simulink model "transmitFullSim2019a"  (R2019a)
settings: Solver=VariableStepAuto  StartTime=0.0  StopTime=0.25  RelTol=1e-3
values from neighbouring files (symbols this model uses):
  Cappr = 5.0616e-11    [transmitData.m]
  Ipr = 2.5055e-7    (= 2.5055e-07)    [transmitData.m]
  Nbps = 4    [transmitData.m]
  Rpr = 45e-3    (= 0.045)    [transmitData.m]
  Ts = 1e-8    (= 1e-08)    [transmitData.m]
libraries: rfports1 x2, commdigbbndam3 x2, commrfcorlib x1, commchan3 x1, commrandsrc3 x1, rftxlines1 x1, commsink2 x1, commutil2 x1, commrflib2 x1
settings Model: Creator=PABLO  LastModifiedBy=marekkulawik

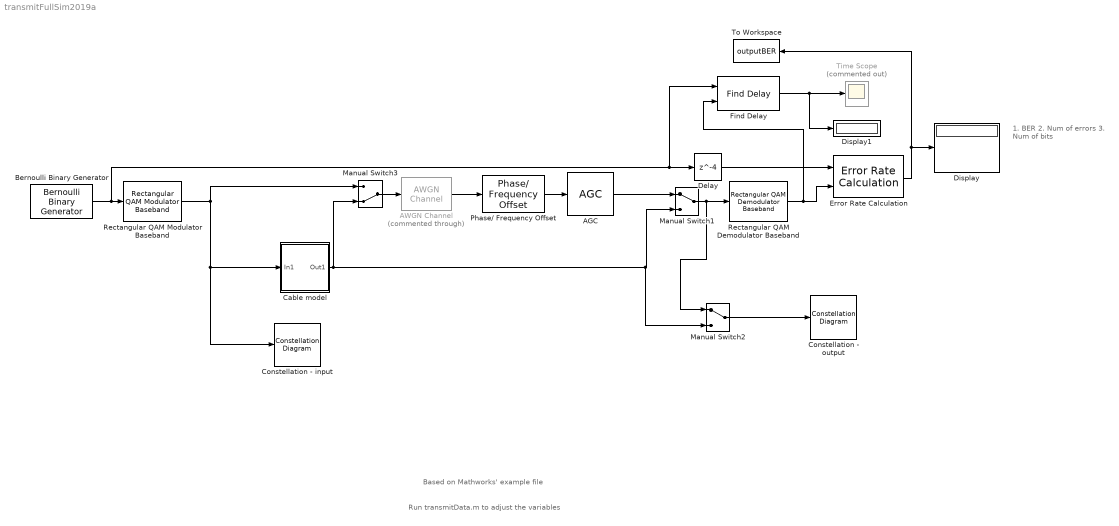
== system transmitFullSim2019a ==
  note: 1. BER
      | 2. Num of errors
      | 3. Num of bits
  note: Run transmitData.m to adjust the variables
  note: Based on Mathworks' example file
  AGC : commrfcorlib/AGC  LegacyMode=off  DetectorMethod=Rectifier  LoopMethod=Linear  UpdatePeriod=100  StepSize=0.1  AdaptationStepSize=0.001  DesiredOutputPower=1  AveragingLength=100  MaximumGain=30  MaxPowerGain=60  GainOutputPort=off  InputPowerOutputPort=off  SimulateUsing=Interpreted execution
      settings: SourceProductName=Communications Toolbox
  AWGN Channel : commchan3/AWGN Channel  Commented=through  InputProcessing=Columns as channels (frame based)  seed=54321  noiseMode="Signal to noise ratio  (SNR)"  EbNodB=EbN0  EsNodB=40  SNRdB=SNR  bitsPerSym=Nbps  Ps=1  Tsym=1e-4*Nbps  variance=1
      settings: SourceProductName=Communications Toolbox
  Bernoulli Binary Generator : commrandsrc3/Bernoulli Binary Generator  ProbabilityOfZero=0.5  SeedSource=Auto  Seed=0  SampleTime=Ts  SamplesPerFrame=Nbps*1  OutputDataType=boolean  SimulateUsing=Interpreted execution
      settings: SourceProductName=Communications Toolbox
  Cable model : Subsystem
  Constellation - input : ConstellationDiagram
  Constellation - output : ConstellationDiagram
  "Delay " : Delay  DelayLength=4  InitialCondition=0
  Display : Display
  Display1 : Display
  Error Rate Calculation : commsink2/Error Rate Calculation  N=0  st_delay=0  cp_mode=Entire frame  subframe=[]  PMode=Port  WsName=ErrorVec  RsMode2=off  stop=on  numErr=tgtMaxErr  maxBits=1e8
      settings: SourceProductName=Communications Toolbox
  Find Delay : commutil2/Find Delay  corrLength=1000  chgSigOP=off  stopUpdate=off  numConstDelay=3
      settings: SourceProductName=Communications Toolbox  SourceProductBaseCode=CM
  Manual Switch1 : ManualSwitch
  Manual Switch2 : ManualSwitch
  Manual Switch3 : ManualSwitch  CurrentSetting=0
  Phase/ Frequency Offset : commrflib2/Phase// Frequency Offset  phaseOffset=270+56.5  freqPort=off  freqOffset=0
      settings: SourceProductName=Communications Toolbox
  Rectangular QAM Demodulator Baseband : commdigbbndam3/Rectangular QAM Demodulator Baseband  M=2^Nbps  OutType=Bit  DecType=Hard decision  VarSource=Dialog  Variance=1  Dec=Binary  Mapping=[0:15]  PowType=Average Power  MinDist=2  AvgPow=1  PeakPow=1  Ph=0  outDtype1=boolean  outDtype2=uint8  derotateFactorWordLen=16  derotateFactorDataTypeStr=Inherit: Same word length as input  derotateFactorLastDataTypeStr=Inherit: Same word length as input  denormFactorWordLen=16  denormFactorDataTypeStr=Inherit: Same word length as input  denormFactorLastDataTypeStr=Inherit: Same word length as input  prodOutWordLen=32  prodOutOverflowMode=Wrap  prodOutRoundingMode=Floor  prodOutOvFlMode=off  prodOutOvFlModeLastStrValue=off  sumWordLen=32
      settings: SourceProductName=Communications Toolbox
  Rectangular QAM Modulator Baseband : commdigbbndam3/Rectangular QAM Modulator Baseband  M=2^Nbps  InType=Bit  Enc=Binary  Mapping=[0:15]  PowType=Average Power  MinDist=2  AvgPow=1  PeakPow=1  Ph=0  outDtype=single  outWordLen=16  outUDDataType=sfix(16)  outFracLenMode=Best precision  outFracLen=15  outDataTypeStr=single  outLastDataTypeStr=single
      settings: SourceProductName=Communications Toolbox
  Time Scope : Scope  Commented=on
  To Workspace : ToWorkspace  VariableName=outputBER  SampleTime=-1
      settings: MaxDataPoints=1  Save2DSignal=2-D array (concatenate along first dimension)
  wires:
  Bernoulli Binary Generator/1 -> Find Delay/1, "Delay "/1, Rectangular QAM Modulator Baseband/1
  Error Rate Calculation/1 -> To Workspace/1, Display/1
  Rectangular QAM Demodulator Baseband/1 -> Find Delay/2, Error Rate Calculation/2
  Rectangular QAM Modulator Baseband/1 -> Cable model/1(In1), Constellation - input/1, Manual Switch3/1
  Manual Switch1/1 -> Manual Switch2/1, Rectangular QAM Demodulator Baseband/1
  Manual Switch2/1 -> Constellation - output/1
  Manual Switch3/1 -> AWGN Channel/1
  AWGN Channel/1 -> Phase/ Frequency Offset/1
  Cable model/1(Out1) -> Manual Switch2/2, Manual Switch1/2, Manual Switch3/2
  Phase/ Frequency Offset/1 -> AGC/1
  AGC/1 -> Manual Switch1/1
  Find Delay/1 -> Display1/1, Time Scope/1
  "Delay "/1 -> Error Rate Calculation/1

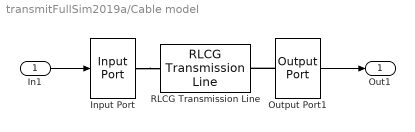
== system transmitFullSim2019a/Cable model ==
  In1 : Inport
  Input Port : rfports1/Input Port  Description=source block  TreatSimulinkInputSignalAs=Source voltage  MaxLength=128  FracBW=0  ModelDelay=0  Fc=2e9  Ts=Nbps*Ts  Zs=50  RFhasDSP=Elements as channels (sample based)  NoiseFlag=off  seed=67987  GoToTag=ACDDBEEHCAIHFUJKVTSPJSL
      settings: SourceProductName=RF Blockset  SourceProductBaseCode=RB
  Output Port1 : rfports1/Output Port  Zl=50  Flag=0  num_Models=0  GoToTag=ACDDBEEHCAIHFUJKVTSPJSL  PlotFreq=User-specified  SourceFreq=Derived from Input Port parameters  Freq=1e9:1e8:3e9  AllPlotType=X-Y plane  AppliedNetworkData=S11  AppliedComplexFormat=Magnitude (decibels)  AppliedNetworkData2=""  AppliedXParameter=Freq  AppliedXFormat=Hz  YOption=Linear  XOption=Linear  PlotZ0=50  DisplayData=off  NoBudgetPlot=Composite data  NetworkData=S11  SmithData=S11  PolarData=S11  ComplexFormat=Magnitude (decibels)  DBFormat=Magnitude (decibels)  DBMFormat=dBm  NoneFormat=None
      settings: SourceProductName=RF Blockset  SourceProductBaseCode=RB
  RLCG Transmission Line : rftxlines1/RLCG Transmission Line  LConnTagsString=__newl0  RConnTagsString=__newr0  R=Rpr  L=Ipr  C=Cappr  G=Conpr  ParamFreq=freq  InterpMethod=Linear  LineLength=length  StubMode=Not a stub  Termination=Open  PlotFreq=User-specified  SourceFreq=User-specified  Freq=[1e9:1.0e6:3e9]  AllPlotType=X-Y plane  AppliedNetworkData=S21  AppliedComplexFormat=Angle (degrees)  AppliedNetworkData2=""  AppliedComplexFormat2=""  AppliedXParameter=Freq  AppliedXFormat=Hz  YOption=Linear  XOption=Linear  PlotZ0=50  DisplayData=off  PlotFreqNoSim=User-specified  NetworkData=S21  SmithData=S11  PolarData=S11  ComplexFormat=Angle  DBFormat=Magnitude (decibels)  NoneFormat=None
      settings: SourceProductName=RF Blockset  SourceProductBaseCode=RB
  Out1 : Outport
  wires:
  In1/1 -> Input Port/1
  Output Port1/1 -> Out1/1
  connections:
  Output Port1/LConn1 -- RLCG Transmission Line/RConn1
  Input Port/RConn1 -- RLCG Transmission Line/LConn1
